simulink model "modelHW4"  (R2023a)
settings: Solver=VariableStepAuto  StartTime=0.0  StopTime=1.5 * Ts  RelTol=1e-3
values from neighbouring files (symbols this model uses):
  A = [0, 1 ... (first row only)    [initHW4.m]    (also in initLab4.m = [0, 1, 0, 0; lab5m.m = [-f1 0;f1 -f2])
  B = [0 ... (first row only)    [initHW4.m]    (also in initLab4.m = [0; (constA .* constD)./(n .* g); 0; constD]; lab5m.m = [beta;0])
  C = [1, 0]    [initHW4.m]    (also in initLab4.m = [1, 0, 0, 0; lab5m.m = [0 1])
  gammaa = 1    [initHW4.m]    (also in lab5m.m)
  K1 = Kd(:,1:n)    [tsd.m]
  K2 = Kd(:,n+1:n+q)    [tsd.m]
  phia = 1    [initHW4.m]    (also in lab5m.m)
  T = min(Ts / (20 * (nOrder + 1)),      pi / (5 * TbetaMax))    [initHW4.m]    (also in initLab4.m = 0.01; lab5m.m = 0.1)
settings Model: Creator=fwah  LastModifiedBy=fwah
settings OptimizationCC: ReuseModelBlockBuffer=off

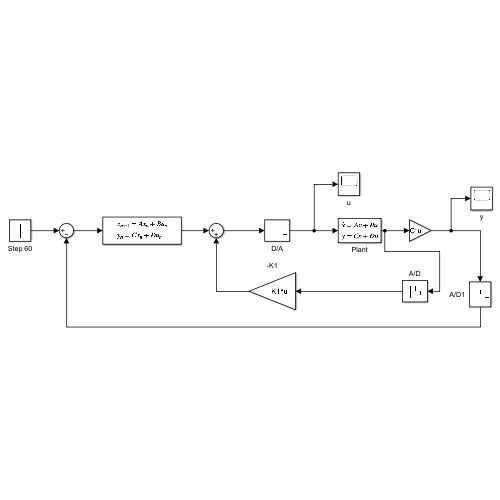
[thumbnail: Simulink's stored preview of the top-level diagram]
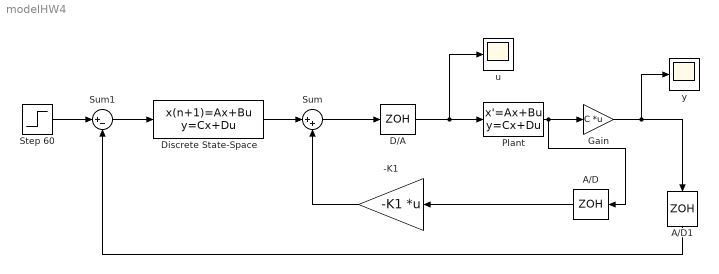
== system modelHW4 ==
  -K1 : Gain  Gain=-K1  Multiplication=Matrix(K*u)
  A/D : ZeroOrderHold  SampleTime=T
  A/D1 : ZeroOrderHold  SampleTime=T
  D/A : ZeroOrderHold  SampleTime=T
  Discrete State-Space : DiscreteStateSpace  A=phia  B=gammaa  C=K2  D=0  SampleTime=T
  Gain : Gain  Gain=C  Multiplication=Matrix(K*u)
  Plant : StateSpace  A=A  B=B  C=eye(2)  D=zeros(2,1)  InitialCondition=0
  Step 60 : Step  Time=0  After=60  SampleTime=0
  Sum : Sum  Inputs=|++
  Sum1 : Sum  Inputs=|+-
  u : Scope
  y : Scope
  wires:
  D/A/1 -> Plant/1, u/1
  Step 60/1 -> Sum1/1
  -K1/1 -> Sum/2
  Sum1/1 -> Discrete State-Space/1
  Discrete State-Space/1 -> Sum/1
  Sum/1 -> D/A/1
  Plant/1 -> A/D/1, Gain/1
  A/D/1 -> -K1/1
  Gain/1 -> A/D1/1, y/1
  A/D1/1 -> Sum1/2
